simulink model "Atomic_Subsystem"  (R2020b)
settings: Solver=FixedStepAuto  StartTime=0.0  StopTime=10.0  FixedStep=0.5  RelTol=1e-3
settings Model: Creator=Puru Gawande  LastModifiedBy=Puru Gawande
settings DataIOCC: SaveOutput=off  SaveTime=off

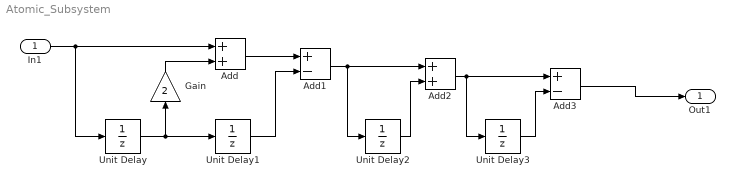
== system Atomic_Subsystem ==
  In1 : Inport  OutDataTypeStr=double  PortDimensions=[1 1]  SampleTime=[0.5,0]
  Add : Sum
  Add1 : Sum  Inputs=+-
  Add2 : Sum
  Add3 : Sum  Inputs=+-
  Gain : Gain  Gain=2
  Unit Delay{,1..3} (4 alike) : UnitDelay  SampleTime=-1  HasFrameUpgradeWarning=on
  Out1 : Outport  OutDataTypeStr=double  PortDimensions=[1 1]  SampleTime=[0.5,0]
  wires:
  Unit Delay/1 -> Gain/1, Unit Delay1/1
  Unit Delay2/1 -> Add2/2
  Add1/1 -> Add2/1, Unit Delay2/1
  Unit Delay1/1 -> Add1/2
  In1/1 -> Unit Delay/1, Add/1
  Gain/1 -> Add/2
  Add/1 -> Add1/1
  Unit Delay3/1 -> Add3/2
  Add2/1 -> Add3/1, Unit Delay3/1
  Add3/1 -> Out1/1
